simulink model "Tarea_31"  (R2020a)
settings: Solver=VariableStepAuto  StartTime=0.0  StopTime=200  RelTol=1e-3
values from neighbouring files (symbols this model uses):
  A = [-3, 2, 0 ... (first row only)    [AsesoriaP3.m]    (also in Circ_Doble_Malla_ODE_plot.m = [0, 1/C2; -1/(R1*C1*R2), -(C2*R1+C2*R2+R1*C1)/(C1*C2*R1*R2)]; ControlThis_P1.m = [-1,-3,0; Controlador_Retro_plot.m = [0, 0, 1, 0; Engranes_ODE_plot.m = [0, 1; -K./(Jm2 + Jm1.*(n2./n1)^2), -B/(Jm2 + Jm1.*(n2./n1)^)
  B = [2, 0 ... (first row only)    [AsesoriaP3.m]    (also in Circ_Doble_Malla_ODE_plot.m = [0; 1/(C1*R1*R2)]; ControlThis_P1.m = [2,4,2; Controlador_Retro_plot.m = [0; Engranes_ODE_plot.m = [0; -1/(n1.*Jm2/2 + n2.*Jm1./n1)])
  C = [0, 3, 0]    [AsesoriaP3.m]    (also in Circ_Doble_Malla_ODE_plot.m = [1 0]; ControlThis_P1.m = [3,2,0; Controlador_Retro_plot.m = [1, 0, 0, 0]; Engranes_ODE_plot.m = [1, 0])
  Dc = [0 ... (first row only)    [Tarea_31.m]
  Fc = 1 / ( C*inv(-A-B*Kc)*B )    [Tarea_31.m]    (also in matlab.mat = 0.394)
  Kc = -[0, 0, 1]*inv(Mc)*Hc    [Tarea_31.m]
  ref = 2*sin(2*t)    [AsesoriaP3.m]    (also in ControlThis_P1.m = 5*tanh(4-t); Ex2_ej1.m = 10 - 2*cos(t); Ex2_ej3.m = 1; Ex3_ej1.m = 1000)
settings Model: Creator=micro microndas  LastModifiedBy=micro microndas

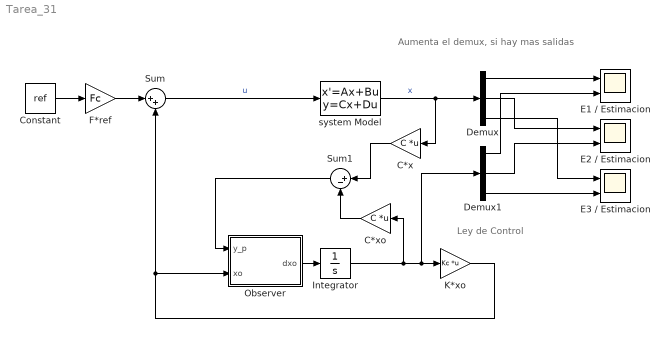
== system Tarea_31 ==
  note: Ley de Control
  note: Aumenta el demux, si hay mas salidas
  C*x : Gain  Gain=C  Multiplication=Matrix(K*u)
  C*xo : Gain  Gain=C  Multiplication=Matrix(K*u)
  Constant : Constant  Value=ref
  Demux : Demux  Outputs=3
  Demux1 : Demux  Outputs=3
  E1 / Estimacion : Scope  NumInputPorts=2
  E2 / Estimacion : Scope  NumInputPorts=2
  E3 / Estimacion : Scope  NumInputPorts=2
  F*ref : Gain  Gain=Fc
  Integrator : Integrator
  K*xo : Gain  Gain=Kc  Multiplication=Matrix(K*u)
  Observer : MATLAB Function  TreatAsAtomicUnit=on
  Sum : Sum  Inputs=|++
  Sum1 : Sum  Inputs=|+-
  system Model : StateSpace  A=A  B=B  C=eye(3)  D=Dc  InitialCondition=[20, 20, 30]
  wires:
  Constant/1 -> F*ref/1
  F*ref/1 -> Sum/1
  Sum/1 -> system Model/1  "u"
  system Model/1 -> C*x/1, Demux/1  "x"
  C*x/1 -> Sum1/1
  Sum1/1 -> Observer/1(y_p)
  Integrator/1 -> C*xo/1, Demux1/1, K*xo/1
  C*xo/1 -> Sum1/2
  Demux/1 -> E1 / Estimacion/1
  Demux1/1 -> E1 / Estimacion/2
  Demux/2 -> E2 / Estimacion/1
  Demux1/2 -> E2 / Estimacion/2
  Demux1/3 -> E3 / Estimacion/2
  Demux/3 -> E3 / Estimacion/1
  Observer/1(dxo) -> Integrator/1
  K*xo/1 -> Observer/2(xo), Sum/2

== matlab function Tarea_31/Observer ==
  data: y_p input; xo input; dxo output
function dxo = fcn(y_p,xo)
ref = 20;
%Polo controlador
Pdc = [-2, -2, -2];
%Polo observador
Pdo = [-4, -4, -4];

A = [0, 0, 2;
     2, 1, -1;
     0, 0, 2];
B = [3;
     0;
     1];
C = [1, 1, 0];

%Ganancias Observador
Mo = [C;
      C*A;
      C*(A^2)];
rank(Mo)
Ho = (A - Pdo(1)*eye(3))*(A - Pdo(2)*eye(3))*(A - Pdo(3)*eye(3));
L = -Ho*inv(Mo)*[0,0,1]';

%Ganancias Controlador
Mc = [B, A*B, (A^2)*B];
rank(Mc)
Hc = (A - Pdc(1)*eye(3))*(A - Pdc(2)*eye(3))*(A - Pdc(3)-eye(3));
Kc = -[0, 0, 1]*inv(Mc)*Hc;
Fc = 1 / ( C*inv(-A-B*Kc)*B );

U = Kc*xo + Fc*ref;

dxo = A*xo + B*U - L*y_p;
